simulink model "I_core_limit"  (R2023b)
settings: configuration reference "slow_tsk_conf" (kept outside this file)
undefined symbols (not defined in the file): nHarmonics, shuntHarmonicsCorrected, shuntMaxRequestedCurrentrms, shuntNumHarmonics
settings Model: DataDictionary=fmuGenerationDictionay.sldd  ModifiedByFormat=Third Equation Ltd  Creator=Third Equation Ltd  LastModifiedBy=Third Equation Ltd
settings ConfigSetRef: SourceName=slow_tsk_conf

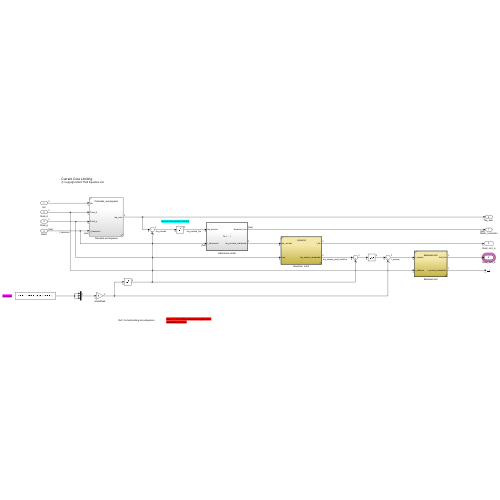
[thumbnail: Simulink's stored preview of the top-level diagram]
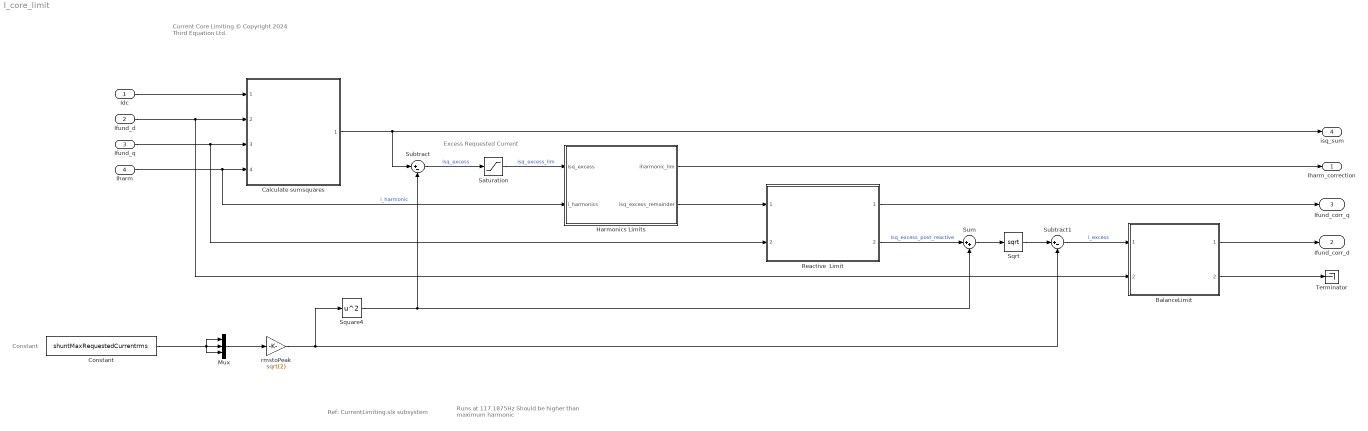
== system I_core_limit ==
  note: Ref: CurrentLimiting.slx subsystem
  note: Current Core Limiting
      | © Copyright 2024 Third Equation Ltd.
  note: Runs at 117.1875Hz Should be higher than
      | maximum harmonic
  note: Excess Requested Current
  note: Constant
  Idc : Inport  OutDataTypeStr=single  PortDimensions=3
  Ifund_d : Inport  Port=2  OutDataTypeStr=single  PortDimensions=3
  Ifund_q : Inport  Port=3  OutDataTypeStr=single  PortDimensions=3
  Iharm : Inport  Port=4  OutDataTypeStr=single  PortDimensions=[3 shuntNumHarmonics]
  BalanceLimit : Subsystem  TreatAsAtomicUnit=on  ReferencedSubsystem=BalanceLimit
  Calculate sumsquares : Subsystem  ReferencedSubsystem=Calculate_sumsquares
  Constant : Constant  Value=shuntMaxRequestedCurrentrms  OutDataTypeStr=single
  Harmonics Limits : Subsystem  TreatAsAtomicUnit=on
  Mux : Mux  Inputs=3
  Reactive  Limit : Subsystem  TreatAsAtomicUnit=on  ReferencedSubsystem=rmsLimit
  Saturation : Saturate  UpperLimit=inf  LowerLimit=0
  Sqrt : Sqrt
  Square4 : Math  Operator=square
  Subtract : Sum  Inputs=|+-
  Subtract1 : Sum  Inputs=|+-
  Sum : Sum  Inputs=|++
  Terminator : Terminator
  rmstoPeak : Gain  Gain=sqrt(2)
  Iharm_correction : Outport  OutDataTypeStr=single  PortDimensions=[3 shuntNumHarmonics]
  Ifund_corr_d : Outport  Port=2  OutDataTypeStr=single  PortDimensions=3
  Ifund_corr_q : Outport  Port=3  OutDataTypeStr=single  PortDimensions=3
  isq_sum : Outport  Port=4  OutDataTypeStr=single  PortDimensions=3
  wires:
  Harmonics Limits/1(iharmonic_lim) -> Iharm_correction/1
  Constant/1 -> Mux/2, Mux/1, Mux/3
  Mux/1 -> rmstoPeak/1
  BalanceLimit/1 -> Ifund_corr_d/1
  Sum/1 -> Sqrt/1
  Sqrt/1 -> Subtract1/1
  Subtract/1 -> Saturation/1  "isq_excess"
  Reactive  Limit/2 -> Sum/1  "isq_excess_post_reactive"
  Square4/1 -> Subtract/2, Sum/2
  Subtract1/1 -> BalanceLimit/1  "i_excess"
  Reactive  Limit/1 -> Ifund_corr_q/1
  Idc/1 -> Calculate sumsquares/1
  rmstoPeak/1 -> Square4/1, Subtract1/2
  Iharm/1 -> Calculate sumsquares/4, Harmonics Limits/2(i_harmonics)  "i_harmonic"
  Ifund_q/1 -> Reactive  Limit/2, Calculate sumsquares/3
  Calculate sumsquares/1 -> Subtract/1, isq_sum/1
  Saturation/1 -> Harmonics Limits/1(isq_excess)  "isq_excess_lim"
  Harmonics Limits/2(isq_excess_remainder) -> Reactive  Limit/1
  BalanceLimit/2 -> Terminator/1
  Ifund_d/1 -> BalanceLimit/2, Calculate sumsquares/2

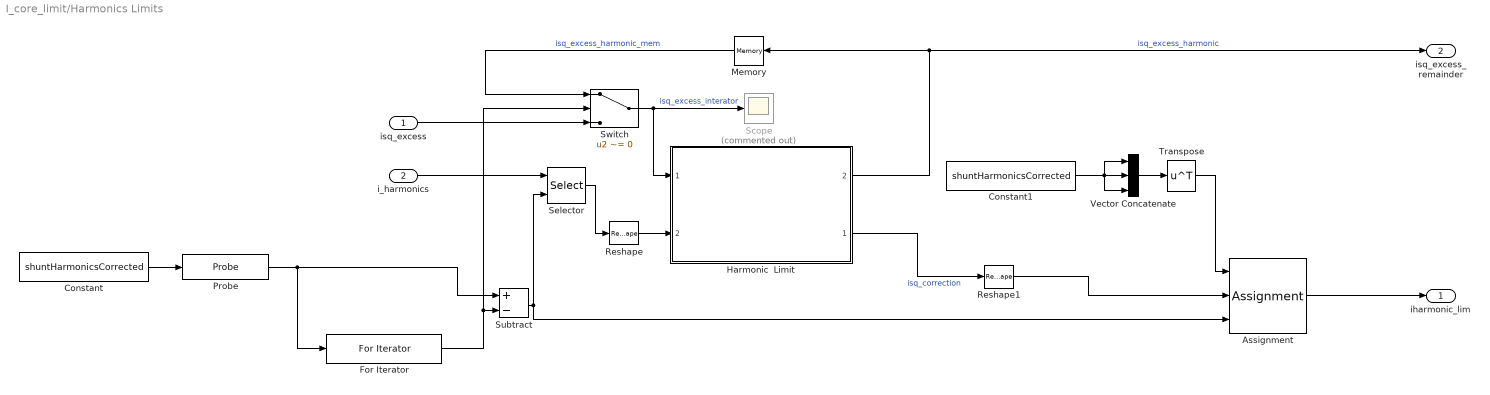
== system I_core_limit/Harmonics Limits ==
  isq_excess : Inport  PortDimensions=3
  i_harmonics : Inport  Port=2  PortDimensions=[3 shuntNumHarmonics]
  Assignment : Assignment  NumberOfDimensions=2  DiagnosticForDimensions=Warning  IndexOptions=Assign all,Index vector (port)  Indices=1,1  OutputSizes=3,nHarmonics
  Constant : Constant  Value=shuntHarmonicsCorrected  OutDataTypeStr=single
  Constant1 : Constant  Value=shuntHarmonicsCorrected  OutDataTypeStr=single
  For Iterator : ForIterator  ResetStates=reset  IterationSource=external  IterationLimit=nHarmonics  IndexMode=Zero-based
  Harmonic  Limit : Subsystem  TreatAsAtomicUnit=on  ReferencedSubsystem=rmsLimit
      settings: PortSchema="{\"entries\":[{\"content\":{\"sides\":[{\"content\":{\"connectorIds\":[\"In1\",\"In2\"]},\"type\":\"ConnectorPlacement.EquallySpacedRectSide\",\"uuid\":\"a0edda42-1093-4dc5-a0fa-0d45baad0397\"},{\"content\":{\"connectorIds\":[\"Out2\",\"Out1\"],\"side\":\"RIGHT\"},\"type\":\"ConnectorPlacement.EquallySpacedRectSide\",\"uuid\":\"9461ca2c-2d49-476d-8dbf-46c4cd226d1a\"},{\"content\":{\"side\":\"TOP\"},\"type\":\"ConnectorPlacement.EquallySpacedRectSide\",\"uuid\":\"ebbd8734-3f86-4c2e-9126-3af595b2078a\"}]},\"type\":\"ConnectorPlacement.EquallySpacedConnector\",\"uuid\":\"3414606b-6b7d-4413-9cd8-bdd988f6d4a8\"}],\"packageUris\":[\"http://schema.mathworks.com/mf0/Connector/R2020b\"],\"version\":\"1.0\"}"
  Memory : Memory  InheritSampleTime=on
  Probe : Probe  ProbeWidth=off  ProbeSampleTime=off  ProbeComplexSignal=off  ProbeSignalDimensions=on  ProbeDimensionsDataType=single
  Reshape : Reshape
  Reshape1 : Reshape  OutputDimensionality=Column vector (2-D)
  Scope : Scope  Commented=on
  Selector : Selector  NumberOfDimensions=2  InputPortWidth=1  IndexOptions=Select all,Index vector (port)  Indices=[1 3],1  OutputSizes=1,1
  Subtract : Sum  Inputs=+-
  Switch : Switch  Criteria=u2 ~= 0  Threshold=1  SaturateOnIntegerOverflow=off  InputSameDT=off
  Transpose : Math  Operator=transpose
  Vector Concatenate : Concatenate  NumInputs=3  Mode=Multidimensional array  ConcatenateDimension=2
  iharmonic_lim : Outport  OutDataTypeStr=single  PortDimensions=[3 shuntNumHarmonics]
  isq_excess_remainder : Outport  Port=2  OutDataTypeStr=single  PortDimensions=3
  wires:
  Transpose/1 -> Assignment/1
  Vector Concatenate/1 -> Transpose/1
  Constant1/1 -> Vector Concatenate/3, Vector Concatenate/1, Vector Concatenate/2
  Constant/1 -> Probe/1
  Reshape1/1 -> Assignment/2
  Reshape/1 -> Harmonic  Limit/2
  Switch/1 -> Scope/1, Harmonic  Limit/1  "isq_excess_interator"
  Harmonic  Limit/2 -> isq_excess_remainder/1, Memory/1  "isq_excess_harmonic"
  Memory/1 -> Switch/1  "isq_excess_harmonic_mem"
  Subtract/1 -> Assignment/3, Selector/2
  For Iterator/1 -> Subtract/2, Switch/2
  Probe/1 -> Subtract/1, For Iterator/1
  Selector/1 -> Reshape/1
  Assignment/1 -> iharmonic_lim/1
  Harmonic  Limit/1 -> Reshape1/1  "isq_correction"
  i_harmonics/1 -> Selector/1
  isq_excess/1 -> Switch/3
